simulink model "model_min_mine"  (R2018a)
settings: Solver=ode45  StartTime=0.0  StopTime=20  RelTol=1e-3
(part 2 of 10)

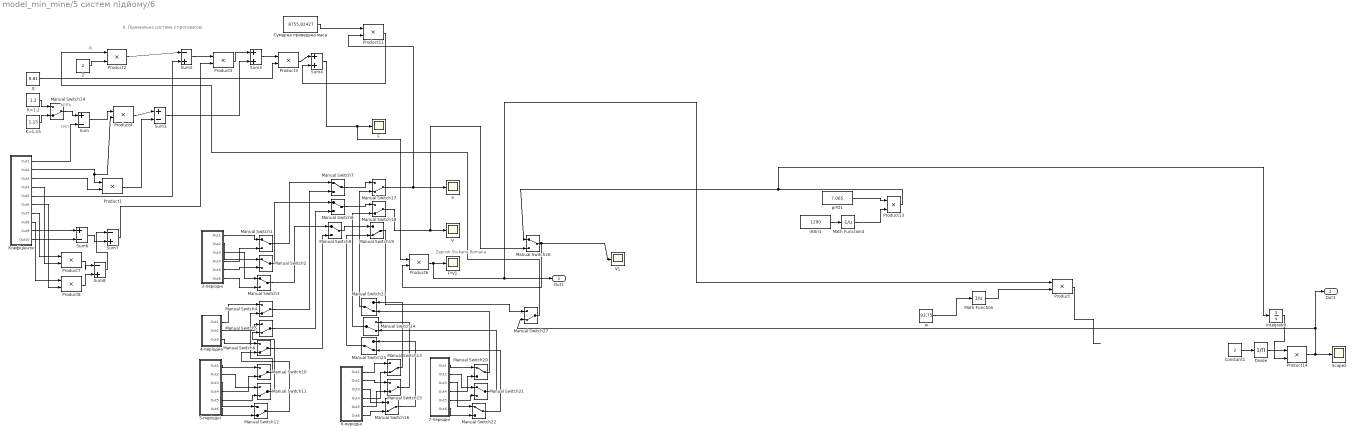
== system model_min_mine/5 систем підйому/6 ==
  note: кліть
  note: скіп
  note: Xi
  note: 6. Піднімальна система з противагою
  note: Zapusk Stukana Romana
  (60i)1 : Constant  Value=1200
  2 : Constant  Value=2
  3-періодні : Subsystem
  "4-періодна " : Subsystem
  5-періодні : Subsystem
  6-періодні : Subsystem
  7-періодні : Subsystem
  Constant1 : Constant  Value=2
  Divide : Product  Inputs=/
  F : Scope
  F*V1 : Scope
  Integrator : Integrator
  K=1.15 : Constant  Value=1.15
  K=1.2 : Constant  Value=1.2
  Manual Switch{1..3,7..9,20..22,26} (10 alike) : ManualSwitch
  Manual Switch{4..6,10..19,23..25,27} (17 alike) : ManualSwitch  CurrentSetting=0
  Math Function : Math  Operator=reciprocal  SaturateOnIntegerOverflow=on
  Math Function4 : Math  Operator=reciprocal  SaturateOnIntegerOverflow=on
  Product{,1..8,11,14} (11 alike) : Product  SaturateOnIntegerOverflow=on  OutDataTypeStr=Inherit: Same as first input
  Product13 : Product  Inputs=3  RndMeth=Zero
  Scope2 : Scope
  Sum : Sum  Inputs=|+-  SaturateOnIntegerOverflow=on
  Sum1 : Sum  Inputs=|+-  SaturateOnIntegerOverflow=on
  Sum2 : Sum  Inputs=|-+  SaturateOnIntegerOverflow=on
  Sum3 : Sum  Inputs=|++  SaturateOnIntegerOverflow=on
  Sum4 : Sum  Inputs=|++  SaturateOnIntegerOverflow=on
  Sum6 : Sum  Inputs=|+-  SaturateOnIntegerOverflow=on
  Sum7 : Sum  Inputs=|-+  SaturateOnIntegerOverflow=on
  Sum8 : Sum  Inputs=|-+  SaturateOnIntegerOverflow=on
  V : Scope
  V1 : Scope
  a : Scope
  g : Constant  Value=9.81
  pi*D1 : Constant  Value=7.065
  w : Constant  Value=93.75
  Коефіцієнти : Subsystem
  Сумарна приведена маса : Constant  Value=8755.82427
  Out1 : Outport
  Out3 : Outport  Port=2
  wires:
  K=1.2/1 -> Manual Switch14/1
  K=1.15/1 -> Manual Switch14/2
  Manual Switch14/1 -> Sum/1
  Коефіцієнти/1(Out1) -> Sum/2
  Sum/1 -> Product4/1
  Коефіцієнти/2(Out2) -> Product4/2, Product1/1
  Коефіцієнти/3(Out3) -> Product1/2
  Product4/1 -> Sum1/1
  Product1/1 -> Sum1/2
  Product2/1 -> Sum2/1
  Коефіцієнти/5(Out5) -> Sum2/2
  Sum1/1 -> Sum3/2
  Sum3/1 -> Product3/1
  g/1 -> Product3/2
  Коефіцієнти/4(Out4) -> Product7/2
  Sum2/1 -> Product5/1
  Product5/1 -> Sum3/1
  Product3/1 -> Sum4/1
  Sum4/1 -> F/1, Product6/1
  2/1 -> Product2/2
  Сумарна приведена маса/1 -> Product11/1
  Product11/1 -> Sum4/2
  Коефіцієнти/6(Out6) -> Product8/2
  Коефіцієнти/9(Out9) -> Sum6/1
  Коефіцієнти/10(Out10) -> Sum6/2
  Sum6/1 -> Sum7/2
  Коефіцієнти/7(Out7) -> Product7/1
  Коефіцієнти/8(Out8) -> Product8/1
  Product8/1 -> Sum8/2
  Product7/1 -> Sum8/1
  Sum8/1 -> Sum7/1
  Sum7/1 -> Product5/2
  Manual Switch25/1 -> Manual Switch19/2
  Manual Switch24/1 -> Manual Switch18/2
  Manual Switch23/1 -> Manual Switch17/2
  Manual Switch16/1 -> Manual Switch25/1
  Manual Switch15/1 -> Manual Switch24/1
  Manual Switch13/1 -> Manual Switch23/1
  Manual Switch22/1 -> Manual Switch25/2
  Manual Switch21/1 -> Manual Switch24/2
  Manual Switch20/1 -> Manual Switch23/2
  Manual Switch8/1 -> Manual Switch18/1
  Manual Switch17/1 -> a/1, Product11/2
  Manual Switch7/1 -> Manual Switch17/1
  Manual Switch12/1 -> Manual Switch6/2
  Manual Switch11/1 -> Manual Switch5/2
  Manual Switch10/1 -> Manual Switch4/2
  Manual Switch6/1 -> Manual Switch9/2
  Manual Switch5/1 -> Manual Switch8/2
  Manual Switch4/1 -> Manual Switch7/2
  Manual Switch9/1 -> Manual Switch19/1
  Manual Switch2/1 -> Manual Switch8/1
  Manual Switch1/1 -> Manual Switch7/1
  Manual Switch3/1 -> Manual Switch9/1
  Product6/1 -> F*V1/1, Out1/1, Product/1
  Manual Switch18/1 -> V/1, Manual Switch26/2
  3-періодні/1(Out1) -> Manual Switch1/1
  3-періодні/2(Out2) -> Manual Switch2/1
  3-періодні/3(Out3) -> Manual Switch3/1
  3-періодні/4(Out4) -> Manual Switch1/2
  3-періодні/5(Out5) -> Manual Switch2/2
  3-періодні/6(Out6) -> Manual Switch3/2
  "4-періодна "/1(Out1) -> Manual Switch4/1
  "4-періодна "/2(Out2) -> Manual Switch5/1
  "4-періодна "/3(Out3) -> Manual Switch6/1
  5-періодні/1(Out1) -> Manual Switch10/1
  5-періодні/2(Out2) -> Manual Switch11/1
  5-періодні/3(Out3) -> Manual Switch12/1
  5-періодні/4(Out4) -> Manual Switch10/2
  5-періодні/5(Out5) -> Manual Switch11/2
  5-періодні/6(Out6) -> Manual Switch12/2
  6-періодні/1(Out1) -> Manual Switch13/1
  6-періодні/2(Out2) -> Manual Switch15/1
  6-періодні/3(Out3) -> Manual Switch16/1
  6-періодні/4(Out4) -> Manual Switch13/2
  6-періодні/5(Out5) -> Manual Switch15/2
  6-періодні/6(Out6) -> Manual Switch16/2
  7-періодні/1(Out1) -> Manual Switch20/1
  7-періодні/2(Out2) -> Manual Switch21/1
  7-періодні/3(Out3) -> Manual Switch22/1
  7-періодні/4(Out4) -> Manual Switch20/2
  7-періодні/5(Out5) -> Manual Switch21/2
  7-періодні/6(Out6) -> Manual Switch22/2
  Product/1 -> ?
  Math Function/1 -> Product/2
  w/1 -> Math Function/1
  Integrator/1 -> Product14/2
  Product14/1 -> Scope2/1, Out3/1, Manual Switch27/2
  Divide/1 -> Product14/1
  Constant1/1 -> Divide/1
  pi*D1/1 -> Product13/1
  (60i)1/1 -> Math Function4/1
  Math Function4/1 -> Product13/3
  Product13/1 -> Manual Switch26/1, Integrator/1
  Manual Switch26/1 -> Product6/2, V1/1
  Manual Switch19/1 -> Manual Switch27/1
  Manual Switch27/1 -> Product2/1

== system model_min_mine/5 систем підйому/1/3-періодні ==
  note: 1. Криволінійна трьохперіодна
  note: a
  note: 2. Пр
  Криволінійна-3 : Subsystem
  Пр : Subsystem
  Out1 : Outport
  Out2 : Outport  Port=2
  Out3 : Outport  Port=3
  Out4 : Outport  Port=4
  Out5 : Outport  Port=5
  Out6 : Outport  Port=6
  wires:
  Криволінійна-3/1(Out1) -> Out1/1
  Криволінійна-3/2(Out2) -> Out2/1
  Криволінійна-3/3(Out3) -> Out3/1
  Пр/1(Out1) -> Out4/1
  Пр/2(Out2) -> Out5/1
  Пр/3(Out3) -> Out6/1

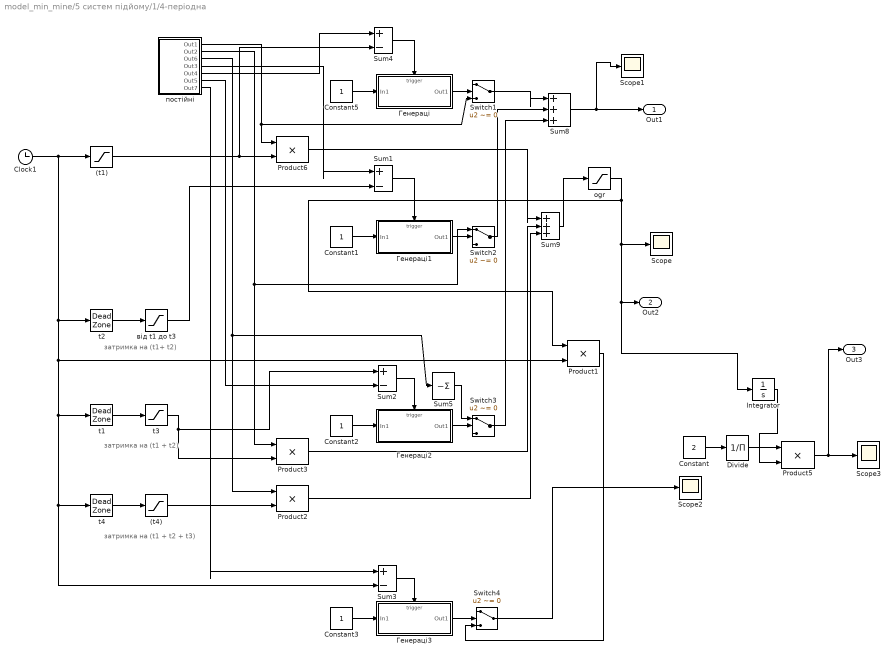
== system model_min_mine/5 систем підйому/1/4-періодна  ==
  note: затримка на
      | (t1 + t2 + t3)
  note: затримка на
      | (t1 + t2)
  note: затримка на
      |  (t1+ t2)
  (t1) : Saturate  UpperLimit=1.15  LowerLimit=0
  (t4) : Saturate  UpperLimit=1  LowerLimit=0
  Clock1 : Clock
  Constant : Constant  Value=2
  Constant{1..3,5} (4 alike) : Constant
  Divide : Product  Inputs=/
  Integrator : Integrator
  Product{1..3,5..6} (5 alike) : Product  SaturateOnIntegerOverflow=on  OutDataTypeStr=Inherit: Same as first input
  Scope{,1..3} (4 alike) : Scope
  Sum{1..4} (4 alike) : Sum  Inputs=|+-  SaturateOnIntegerOverflow=on
  Sum5 : Sum  Inputs=|-  SaturateOnIntegerOverflow=on
  Sum8 : Sum  Inputs=|+++  SaturateOnIntegerOverflow=on
  Sum9 : Sum  Inputs=|+++  SaturateOnIntegerOverflow=on
  Switch{1..4} (4 alike) : Switch  Criteria=u2 ~= 0  RndMeth=Zero  SaturateOnIntegerOverflow=on
  ogr : Saturate  UpperLimit=100  LowerLimit=0
  t1 : DeadZone  LowerValue=0  UpperValue=6.15  SaturateOnIntegerOverflow=on
  t2 : DeadZone  LowerValue=0  UpperValue=3.15  SaturateOnIntegerOverflow=on
  t3 : Saturate  UpperLimit=2  LowerLimit=0
  t4 : DeadZone  LowerValue=0  UpperValue=7.15  SaturateOnIntegerOverflow=on
  Генераці : Subsystem  TreatAsAtomicUnit=on
  Генераці1 : Subsystem  TreatAsAtomicUnit=on
  Генераці2 : Subsystem  TreatAsAtomicUnit=on
  Генераці3 : Subsystem  TreatAsAtomicUnit=on
  від t1 до t3 : Saturate  UpperLimit=3  LowerLimit=0
  постійні : Subsystem
  Out1 : Outport
  Out2 : Outport  Port=2
  Out3 : Outport  Port=3
  wires:
  (t4)/1 -> Product2/2
  t4/1 -> (t4)/1
  Product6/1 -> Sum9/1
  Product2/1 -> Sum9/3
  Product3/1 -> Sum9/2
  ogr/1 -> Product1/1, Scope/1, Out2/1, Integrator/1
  Sum5/1 -> Switch3/1
  від t1 до t3/1 -> Sum1/2
  Product1/1 -> Switch4/3
  Switch4/1 -> Scope2/1
  Генераці3/1(Out1) -> Switch4/2
  Sum3/1 -> Генераці3/Trigger
  Constant3/1 -> Генераці3/1(In1)
  постійні/7(Out7) -> Sum3/1
  t3/1 -> Product3/2, Sum2/1
  t1/1 -> t3/1
  постійні/6(Out5) -> Sum2/2
  Switch3/1 -> Sum8/3
  постійні/3(Out6) -> Sum5/1, Product2/1
  Constant2/1 -> Генераці2/1(In1)
  Sum2/1 -> Генераці2/Trigger
  Генераці2/1(Out1) -> Switch3/2
  постійні/1(Out1) -> Product6/1, Switch1/3
  t2/1 -> від t1 до t3/1
  Clock1/1 -> (t1)/1, t2/1, Product1/2, t1/1, Sum3/2, t4/1
  (t1)/1 -> Product6/2, Sum4/2
  постійні/2(Out2) -> Switch2/1, Product3/1
  Sum9/1 -> ogr/1
  Constant5/1 -> Генераці/1(In1)
  Sum4/1 -> Генераці/Trigger
  Генераці/1(Out1) -> Switch1/2
  Switch1/1 -> Sum8/1
  постійні/5(Out4) -> Sum4/1
  Constant1/1 -> Генераці1/1(In1)
  Sum1/1 -> Генераці1/Trigger
  Генераці1/1(Out1) -> Switch2/2
  постійні/4(Out3) -> Sum1/1
  Switch2/1 -> Sum8/2
  Sum8/1 -> Out1/1, Scope1/1
  Integrator/1 -> Product5/2
  Product5/1 -> Scope3/1, Out3/1
  Divide/1 -> Product5/1
  Constant/1 -> Divide/1

== system model_min_mine/5 систем підйому/1/5-періодні ==
  криво : Subsystem
  пр : Subsystem
  Out1 : Outport
  Out2 : Outport  Port=2
  Out3 : Outport  Port=3
  Out4 : Outport  Port=4
  Out5 : Outport  Port=5
  Out6 : Outport  Port=6
  wires:
  криво/1(Out1) -> Out1/1
  криво/2(Out2) -> Out2/1
  криво/3(Out3) -> Out3/1
  пр/1(Out1) -> Out4/1
  пр/2(Out2) -> Out5/1
  пр/3(Out3) -> Out6/1

== system model_min_mine/5 систем підйому/1/6-періодні ==
  6-ти періодна криволінійна : Subsystem
  6-ти періодна пр : Subsystem
  Out1 : Outport
  Out2 : Outport  Port=2
  Out3 : Outport  Port=3
  Out4 : Outport  Port=4
  Out5 : Outport  Port=5
  Out6 : Outport  Port=6
  wires:
  6-ти періодна криволінійна/1(Out1) -> Out1/1
  6-ти періодна криволінійна/2(Out2) -> Out2/1
  6-ти періодна криволінійна/3(Out3) -> Out3/1
  6-ти періодна пр/1(Out1) -> Out4/1
  6-ти періодна пр/2(Out2) -> Out5/1
  6-ти періодна пр/3(Out3) -> Out6/1

== system model_min_mine/5 систем підйому/1/7-періодні ==
  7-ми періодна криволінійна : Subsystem
  7-ми періодна пр : Subsystem
  Out1 : Outport
  Out2 : Outport  Port=2
  Out3 : Outport  Port=3
  Out4 : Outport  Port=4
  Out5 : Outport  Port=5
  Out6 : Outport  Port=6
  wires:
  7-ми періодна пр/1(Out1) -> Out1/1
  7-ми періодна пр/2(Out2) -> Out2/1
  7-ми періодна пр/3(Out3) -> Out3/1
  7-ми періодна криволінійна/1(Out1) -> Out4/1
  7-ми періодна криволінійна/2(Out2) -> Out5/1
  7-ми періодна криволінійна/3(Out3) -> Out6/1

== system model_min_mine/5 систем підйому/1/Коефіцієнти ==
  alfa : Constant  Value=1.15
  beta : Constant  Value=1.2
  m вантажу : Constant  Value=1000
  mк : Constant  Value=35
  "Висота стволу - Н, м" : Constant  Value=500
  Out1 : Outport
  Out2 : Outport  Port=2
  Out3 : Outport  Port=3
  Out4 : Outport  Port=4
  Out5 : Outport  Port=5
  wires:
  beta/1 -> Out1/1
  m вантажу/1 -> Out2/1
  alfa/1 -> Out3/1
  mк/1 -> Out4/1
  "Висота стволу - Н, м"/1 -> Out5/1

== system model_min_mine/5 систем підйому/2/3-періодні ==
  note: 1. Криволінійна трьохперіодна
  note: a
  note: 2. Пр
  Криволінійна-3 : Subsystem
  Пр : Subsystem
  Out1 : Outport
  Out2 : Outport  Port=2
  Out3 : Outport  Port=3
  Out4 : Outport  Port=4
  Out5 : Outport  Port=5
  Out6 : Outport  Port=6
  wires:
  Криволінійна-3/1(Out1) -> Out1/1
  Криволінійна-3/2(Out2) -> Out2/1
  Криволінійна-3/3(Out3) -> Out3/1
  Пр/1(Out1) -> Out4/1
  Пр/2(Out2) -> Out5/1
  Пр/3(Out3) -> Out6/1

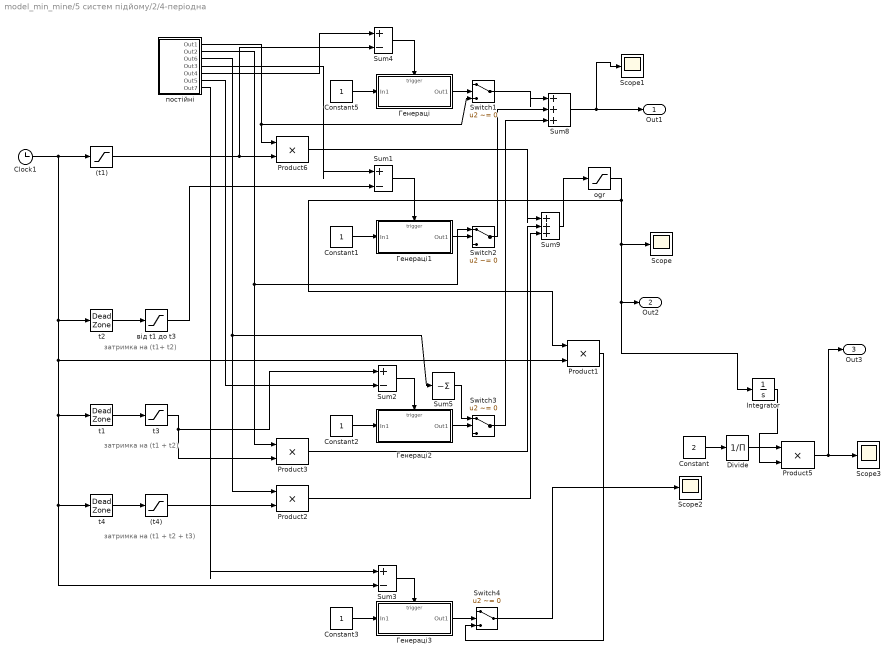
== system model_min_mine/5 систем підйому/2/4-періодна  ==
  note: затримка на
      | (t1 + t2 + t3)
  note: затримка на
      | (t1 + t2)
  note: затримка на
      |  (t1+ t2)
  (t1) : Saturate  UpperLimit=1.15  LowerLimit=0
  (t4) : Saturate  UpperLimit=1  LowerLimit=0
  Clock1 : Clock
  Constant : Constant  Value=2
  Constant{1..3,5} (4 alike) : Constant
  Divide : Product  Inputs=/
  Integrator : Integrator
  Product{1..3,5..6} (5 alike) : Product  SaturateOnIntegerOverflow=on  OutDataTypeStr=Inherit: Same as first input
  Scope{,1..3} (4 alike) : Scope
  Sum{1..4} (4 alike) : Sum  Inputs=|+-  SaturateOnIntegerOverflow=on
  Sum5 : Sum  Inputs=|-  SaturateOnIntegerOverflow=on
  Sum8 : Sum  Inputs=|+++  SaturateOnIntegerOverflow=on
  Sum9 : Sum  Inputs=|+++  SaturateOnIntegerOverflow=on
  Switch{1..4} (4 alike) : Switch  Criteria=u2 ~= 0  RndMeth=Zero  SaturateOnIntegerOverflow=on
  ogr : Saturate  UpperLimit=100  LowerLimit=0
  t1 : DeadZone  LowerValue=0  UpperValue=6.15  SaturateOnIntegerOverflow=on
  t2 : DeadZone  LowerValue=0  UpperValue=3.15  SaturateOnIntegerOverflow=on
  t3 : Saturate  UpperLimit=2  LowerLimit=0
  t4 : DeadZone  LowerValue=0  UpperValue=7.15  SaturateOnIntegerOverflow=on
  Генераці : Subsystem  TreatAsAtomicUnit=on
  Генераці1 : Subsystem  TreatAsAtomicUnit=on
  Генераці2 : Subsystem  TreatAsAtomicUnit=on
  Генераці3 : Subsystem  TreatAsAtomicUnit=on
  від t1 до t3 : Saturate  UpperLimit=3  LowerLimit=0
  постійні : Subsystem
  Out1 : Outport
  Out2 : Outport  Port=2
  Out3 : Outport  Port=3
  wires:
  (t4)/1 -> Product2/2
  t4/1 -> (t4)/1
  Product6/1 -> Sum9/1
  Product2/1 -> Sum9/3
  Product3/1 -> Sum9/2
  ogr/1 -> Product1/1, Scope/1, Out2/1, Integrator/1
  Sum5/1 -> Switch3/1
  від t1 до t3/1 -> Sum1/2
  Product1/1 -> Switch4/3
  Switch4/1 -> Scope2/1
  Генераці3/1(Out1) -> Switch4/2
  Sum3/1 -> Генераці3/Trigger
  Constant3/1 -> Генераці3/1(In1)
  постійні/7(Out7) -> Sum3/1
  t3/1 -> Product3/2, Sum2/1
  t1/1 -> t3/1
  постійні/6(Out5) -> Sum2/2
  Switch3/1 -> Sum8/3
  постійні/3(Out6) -> Sum5/1, Product2/1
  Constant2/1 -> Генераці2/1(In1)
  Sum2/1 -> Генераці2/Trigger
  Генераці2/1(Out1) -> Switch3/2
  постійні/1(Out1) -> Product6/1, Switch1/3
  t2/1 -> від t1 до t3/1
  Clock1/1 -> (t1)/1, t2/1, Product1/2, t1/1, Sum3/2, t4/1
  (t1)/1 -> Product6/2, Sum4/2
  постійні/2(Out2) -> Switch2/1, Product3/1
  Sum9/1 -> ogr/1
  Constant5/1 -> Генераці/1(In1)
  Sum4/1 -> Генераці/Trigger
  Генераці/1(Out1) -> Switch1/2
  Switch1/1 -> Sum8/1
  постійні/5(Out4) -> Sum4/1
  Constant1/1 -> Генераці1/1(In1)
  Sum1/1 -> Генераці1/Trigger
  Генераці1/1(Out1) -> Switch2/2
  постійні/4(Out3) -> Sum1/1
  Switch2/1 -> Sum8/2
  Sum8/1 -> Out1/1, Scope1/1
  Integrator/1 -> Product5/2
  Product5/1 -> Scope3/1, Out3/1
  Divide/1 -> Product5/1
  Constant/1 -> Divide/1

== system model_min_mine/5 систем підйому/2/5-періодні ==
  криво : Subsystem
  пр : Subsystem
  Out1 : Outport
  Out2 : Outport  Port=2
  Out3 : Outport  Port=3
  Out4 : Outport  Port=4
  Out5 : Outport  Port=5
  Out6 : Outport  Port=6
  wires:
  криво/1(Out1) -> Out1/1
  криво/2(Out2) -> Out2/1
  криво/3(Out3) -> Out3/1
  пр/1(Out1) -> Out4/1
  пр/2(Out2) -> Out5/1
  пр/3(Out3) -> Out6/1

== system model_min_mine/5 систем підйому/2/6-періодні ==
  6-ти періодна криволінійна : Subsystem
  6-ти періодна пр : Subsystem
  Out1 : Outport
  Out2 : Outport  Port=2
  Out3 : Outport  Port=3
  Out4 : Outport  Port=4
  Out5 : Outport  Port=5
  Out6 : Outport  Port=6
  wires:
  6-ти періодна криволінійна/1(Out1) -> Out1/1
  6-ти періодна криволінійна/2(Out2) -> Out2/1
  6-ти періодна криволінійна/3(Out3) -> Out3/1
  6-ти періодна пр/1(Out1) -> Out4/1
  6-ти періодна пр/2(Out2) -> Out5/1
  6-ти періодна пр/3(Out3) -> Out6/1

== system model_min_mine/5 систем підйому/2/7-періодні ==
  7-ми періодна криволінійна : Subsystem
  7-ми періодна пр : Subsystem
  Out1 : Outport
  Out2 : Outport  Port=2
  Out3 : Outport  Port=3
  Out4 : Outport  Port=4
  Out5 : Outport  Port=5
  Out6 : Outport  Port=6
  wires:
  7-ми періодна пр/1(Out1) -> Out1/1
  7-ми періодна пр/2(Out2) -> Out2/1
  7-ми періодна пр/3(Out3) -> Out3/1
  7-ми періодна криволінійна/1(Out1) -> Out4/1
  7-ми періодна криволінійна/2(Out2) -> Out5/1
  7-ми періодна криволінійна/3(Out3) -> Out6/1

== system model_min_mine/5 систем підйому/2/Коефіцієнти ==
  alfa : Constant  Value=1.15
  beta : Constant  Value=1.2
  m вантажу : Constant  Value=1000
  Out1 : Outport
  Out2 : Outport  Port=2
  Out3 : Outport  Port=3
  wires:
  beta/1 -> Out1/1
  m вантажу/1 -> Out2/1
  alfa/1 -> Out3/1

== system model_min_mine/5 систем підйому/3/3-періодні ==
  note: 1. Криволінійна трьохперіодна
  note: a
  note: 2. Пр
  Криволінійна-3 : Subsystem
  Пр : Subsystem
  Out1 : Outport
  Out2 : Outport  Port=2
  Out3 : Outport  Port=3
  Out4 : Outport  Port=4
  Out5 : Outport  Port=5
  Out6 : Outport  Port=6
  wires:
  Криволінійна-3/1(Out1) -> Out1/1
  Криволінійна-3/2(Out2) -> Out2/1
  Криволінійна-3/3(Out3) -> Out3/1
  Пр/1(Out1) -> Out4/1
  Пр/2(Out2) -> Out5/1
  Пр/3(Out3) -> Out6/1

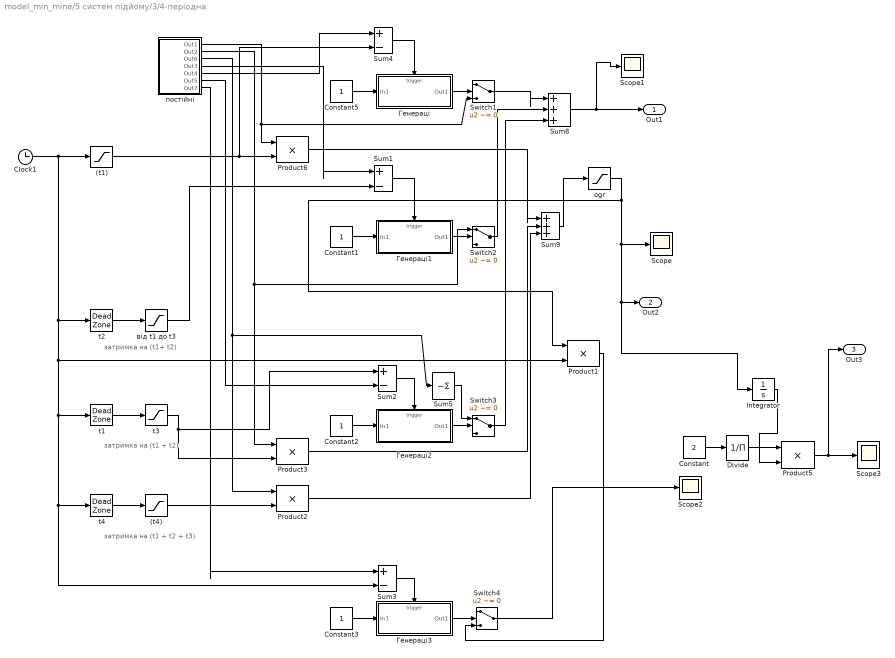
== system model_min_mine/5 систем підйому/3/4-періодна  ==
  note: затримка на
      | (t1 + t2 + t3)
  note: затримка на
      | (t1 + t2)
  note: затримка на
      |  (t1+ t2)
  (t1) : Saturate  UpperLimit=1.15  LowerLimit=0
  (t4) : Saturate  UpperLimit=1  LowerLimit=0
  Clock1 : Clock
  Constant : Constant  Value=2
  Constant{1..3,5} (4 alike) : Constant
  Divide : Product  Inputs=/
  Integrator : Integrator
  Product{1..3,5..6} (5 alike) : Product  SaturateOnIntegerOverflow=on  OutDataTypeStr=Inherit: Same as first input
  Scope{,1..3} (4 alike) : Scope
  Sum{1..4} (4 alike) : Sum  Inputs=|+-  SaturateOnIntegerOverflow=on
  Sum5 : Sum  Inputs=|-  SaturateOnIntegerOverflow=on
  Sum8 : Sum  Inputs=|+++  SaturateOnIntegerOverflow=on
  Sum9 : Sum  Inputs=|+++  SaturateOnIntegerOverflow=on
  Switch{1..4} (4 alike) : Switch  Criteria=u2 ~= 0  RndMeth=Zero  SaturateOnIntegerOverflow=on
  ogr : Saturate  UpperLimit=100  LowerLimit=0
  t1 : DeadZone  LowerValue=0  UpperValue=6.15  SaturateOnIntegerOverflow=on
  t2 : DeadZone  LowerValue=0  UpperValue=3.15  SaturateOnIntegerOverflow=on
  t3 : Saturate  UpperLimit=2  LowerLimit=0
  t4 : DeadZone  LowerValue=0  UpperValue=7.15  SaturateOnIntegerOverflow=on
  Генераці : Subsystem  TreatAsAtomicUnit=on
  Генераці1 : Subsystem  TreatAsAtomicUnit=on
  Генераці2 : Subsystem  TreatAsAtomicUnit=on
  Генераці3 : Subsystem  TreatAsAtomicUnit=on
  від t1 до t3 : Saturate  UpperLimit=3  LowerLimit=0
  постійні : Subsystem
  Out1 : Outport
  Out2 : Outport  Port=2
  Out3 : Outport  Port=3
  wires:
  (t4)/1 -> Product2/2
  t4/1 -> (t4)/1
  Product6/1 -> Sum9/1
  Product2/1 -> Sum9/3
  Product3/1 -> Sum9/2
  ogr/1 -> Product1/1, Scope/1, Out2/1, Integrator/1
  Sum5/1 -> Switch3/1
  від t1 до t3/1 -> Sum1/2
  Product1/1 -> Switch4/3
  Switch4/1 -> Scope2/1
  Генераці3/1(Out1) -> Switch4/2
  Sum3/1 -> Генераці3/Trigger
  Constant3/1 -> Генераці3/1(In1)
  постійні/7(Out7) -> Sum3/1
  t3/1 -> Product3/2, Sum2/1
  t1/1 -> t3/1
  постійні/6(Out5) -> Sum2/2
  Switch3/1 -> Sum8/3
  постійні/3(Out6) -> Sum5/1, Product2/1
  Constant2/1 -> Генераці2/1(In1)
  Sum2/1 -> Генераці2/Trigger
  Генераці2/1(Out1) -> Switch3/2
  постійні/1(Out1) -> Product6/1, Switch1/3
  t2/1 -> від t1 до t3/1
  Clock1/1 -> (t1)/1, t2/1, Product1/2, t1/1, Sum3/2, t4/1
  (t1)/1 -> Product6/2, Sum4/2
  постійні/2(Out2) -> Switch2/1, Product3/1
  Sum9/1 -> ogr/1
  Constant5/1 -> Генераці/1(In1)
  Sum4/1 -> Генераці/Trigger
  Генераці/1(Out1) -> Switch1/2
  Switch1/1 -> Sum8/1
  постійні/5(Out4) -> Sum4/1
  Constant1/1 -> Генераці1/1(In1)
  Sum1/1 -> Генераці1/Trigger
  Генераці1/1(Out1) -> Switch2/2
  постійні/4(Out3) -> Sum1/1
  Switch2/1 -> Sum8/2
  Sum8/1 -> Out1/1, Scope1/1
  Integrator/1 -> Product5/2
  Product5/1 -> Scope3/1, Out3/1
  Divide/1 -> Product5/1
  Constant/1 -> Divide/1

== system model_min_mine/5 систем підйому/3/5-періодні ==
  криво : Subsystem
  пр : Subsystem
  Out1 : Outport
  Out2 : Outport  Port=2
  Out3 : Outport  Port=3
  Out4 : Outport  Port=4
  Out5 : Outport  Port=5
  Out6 : Outport  Port=6
  wires:
  криво/1(Out1) -> Out1/1
  криво/2(Out2) -> Out2/1
  криво/3(Out3) -> Out3/1
  пр/1(Out1) -> Out4/1
  пр/2(Out2) -> Out5/1
  пр/3(Out3) -> Out6/1

== system model_min_mine/5 систем підйому/3/6-періодні ==
  6-ти періодна криволінійна : Subsystem
  6-ти періодна пр : Subsystem
  Out1 : Outport
  Out2 : Outport  Port=2
  Out3 : Outport  Port=3
  Out4 : Outport  Port=4
  Out5 : Outport  Port=5
  Out6 : Outport  Port=6
  wires:
  6-ти періодна криволінійна/1(Out1) -> Out1/1
  6-ти періодна криволінійна/2(Out2) -> Out2/1
  6-ти періодна криволінійна/3(Out3) -> Out3/1
  6-ти періодна пр/1(Out1) -> Out4/1
  6-ти періодна пр/2(Out2) -> Out5/1
  6-ти періодна пр/3(Out3) -> Out6/1

== system model_min_mine/5 систем підйому/3/7-періодні ==
  7-ми періодна криволінійна : Subsystem
  7-ми періодна пр : Subsystem
  Out1 : Outport
  Out2 : Outport  Port=2
  Out3 : Outport  Port=3
  Out4 : Outport  Port=4
  Out5 : Outport  Port=5
  Out6 : Outport  Port=6
  wires:
  7-ми періодна пр/1(Out1) -> Out1/1
  7-ми періодна пр/2(Out2) -> Out2/1
  7-ми періодна пр/3(Out3) -> Out3/1
  7-ми періодна криволінійна/1(Out1) -> Out4/1
  7-ми періодна криволінійна/2(Out2) -> Out5/1
  7-ми періодна криволінійна/3(Out3) -> Out6/1

== system model_min_mine/5 систем підйому/3/Коефіцієнти ==
  alfa : Constant  Value=1.15
  beta : Constant  Value=1.2
  m вантажу : Constant  Value=1000
  mк : Constant  Value=35
  "mк/ " : Constant  Value=45
  "Висота стволу - Н, м" : Constant  Value=500
  Out1 : Outport
  Out2 : Outport  Port=2
  Out3 : Outport  Port=3
  Out4 : Outport  Port=4
  Out5 : Outport  Port=5
  Out6 : Outport  Port=6
  wires:
  beta/1 -> Out1/1
  m вантажу/1 -> Out2/1
  alfa/1 -> Out3/1
  mк/1 -> Out4/1
  "Висота стволу - Н, м"/1 -> Out5/1
  "mк/ "/1 -> Out6/1

== system model_min_mine/5 систем підйому/4/3-періодні ==
  note: 1. Криволінійна трьохперіодна
  note: a
  note: 2. Пр
  Криволінійна-3 : Subsystem
  Пр : Subsystem
  Out1 : Outport
  Out2 : Outport  Port=2
  Out3 : Outport  Port=3
  Out4 : Outport  Port=4
  Out5 : Outport  Port=5
  Out6 : Outport  Port=6
  wires:
  Криволінійна-3/1(Out1) -> Out1/1
  Криволінійна-3/2(Out2) -> Out2/1
  Криволінійна-3/3(Out3) -> Out3/1
  Пр/1(Out1) -> Out4/1
  Пр/2(Out2) -> Out5/1
  Пр/3(Out3) -> Out6/1

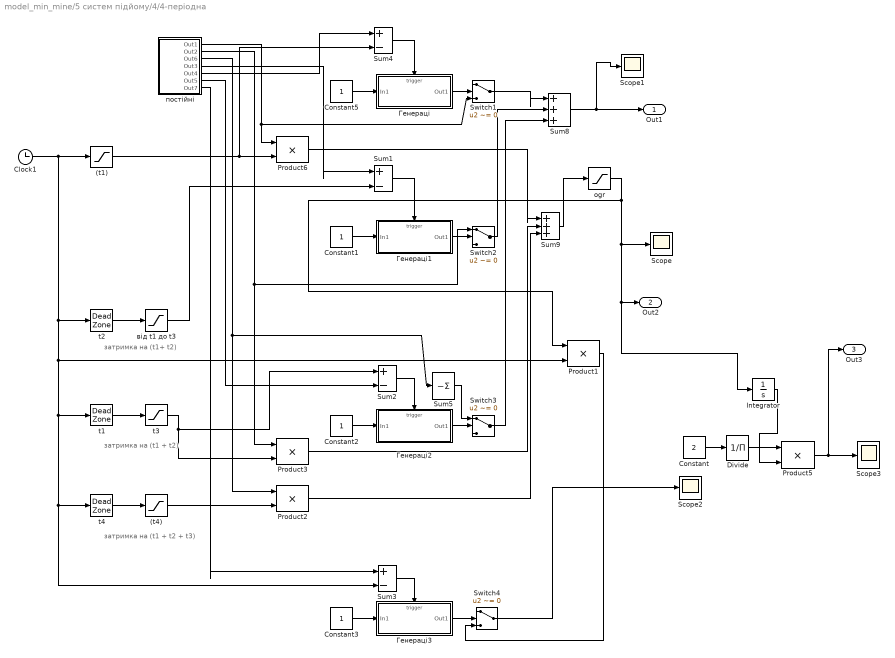
== system model_min_mine/5 систем підйому/4/4-періодна  ==
  note: затримка на
      | (t1 + t2 + t3)
  note: затримка на
      | (t1 + t2)
  note: затримка на
      |  (t1+ t2)
  (t1) : Saturate  UpperLimit=1.15  LowerLimit=0
  (t4) : Saturate  UpperLimit=1  LowerLimit=0
  Clock1 : Clock
  Constant : Constant  Value=2
  Constant{1..3,5} (4 alike) : Constant
  Divide : Product  Inputs=/
  Integrator : Integrator
  Product{1..3,5..6} (5 alike) : Product  SaturateOnIntegerOverflow=on  OutDataTypeStr=Inherit: Same as first input
  Scope{,1..3} (4 alike) : Scope
  Sum{1..4} (4 alike) : Sum  Inputs=|+-  SaturateOnIntegerOverflow=on
  Sum5 : Sum  Inputs=|-  SaturateOnIntegerOverflow=on
  Sum8 : Sum  Inputs=|+++  SaturateOnIntegerOverflow=on
  Sum9 : Sum  Inputs=|+++  SaturateOnIntegerOverflow=on
  Switch{1..4} (4 alike) : Switch  Criteria=u2 ~= 0  RndMeth=Zero  SaturateOnIntegerOverflow=on
  ogr : Saturate  UpperLimit=100  LowerLimit=0
  t1 : DeadZone  LowerValue=0  UpperValue=6.15  SaturateOnIntegerOverflow=on
  t2 : DeadZone  LowerValue=0  UpperValue=3.15  SaturateOnIntegerOverflow=on
  t3 : Saturate  UpperLimit=2  LowerLimit=0
  t4 : DeadZone  LowerValue=0  UpperValue=7.15  SaturateOnIntegerOverflow=on
  Генераці : Subsystem  TreatAsAtomicUnit=on
  Генераці1 : Subsystem  TreatAsAtomicUnit=on
  Генераці2 : Subsystem  TreatAsAtomicUnit=on
  Генераці3 : Subsystem  TreatAsAtomicUnit=on
  від t1 до t3 : Saturate  UpperLimit=3  LowerLimit=0
  постійні : Subsystem
  Out1 : Outport
  Out2 : Outport  Port=2
  Out3 : Outport  Port=3
  wires:
  (t4)/1 -> Product2/2
  t4/1 -> (t4)/1
  Product6/1 -> Sum9/1
  Product2/1 -> Sum9/3
  Product3/1 -> Sum9/2
  ogr/1 -> Product1/1, Scope/1, Out2/1, Integrator/1
  Sum5/1 -> Switch3/1
  від t1 до t3/1 -> Sum1/2
  Product1/1 -> Switch4/3
  Switch4/1 -> Scope2/1
  Генераці3/1(Out1) -> Switch4/2
  Sum3/1 -> Генераці3/Trigger
  Constant3/1 -> Генераці3/1(In1)
  постійні/7(Out7) -> Sum3/1
  t3/1 -> Product3/2, Sum2/1
  t1/1 -> t3/1
  постійні/6(Out5) -> Sum2/2
  Switch3/1 -> Sum8/3
  постійні/3(Out6) -> Sum5/1, Product2/1
  Constant2/1 -> Генераці2/1(In1)
  Sum2/1 -> Генераці2/Trigger
  Генераці2/1(Out1) -> Switch3/2
  постійні/1(Out1) -> Product6/1, Switch1/3
  t2/1 -> від t1 до t3/1
  Clock1/1 -> (t1)/1, t2/1, Product1/2, t1/1, Sum3/2, t4/1
  (t1)/1 -> Product6/2, Sum4/2
  постійні/2(Out2) -> Switch2/1, Product3/1
  Sum9/1 -> ogr/1
  Constant5/1 -> Генераці/1(In1)
  Sum4/1 -> Генераці/Trigger
  Генераці/1(Out1) -> Switch1/2
  Switch1/1 -> Sum8/1
  постійні/5(Out4) -> Sum4/1
  Constant1/1 -> Генераці1/1(In1)
  Sum1/1 -> Генераці1/Trigger
  Генераці1/1(Out1) -> Switch2/2
  постійні/4(Out3) -> Sum1/1
  Switch2/1 -> Sum8/2
  Sum8/1 -> Out1/1, Scope1/1
  Integrator/1 -> Product5/2
  Product5/1 -> Scope3/1, Out3/1
  Divide/1 -> Product5/1
  Constant/1 -> Divide/1

== system model_min_mine/5 систем підйому/4/5-періодні ==
  криво : Subsystem
  пр : Subsystem
  Out1 : Outport
  Out2 : Outport  Port=2
  Out3 : Outport  Port=3
  Out4 : Outport  Port=4
  Out5 : Outport  Port=5
  Out6 : Outport  Port=6
  wires:
  криво/1(Out1) -> Out1/1
  криво/2(Out2) -> Out2/1
  криво/3(Out3) -> Out3/1
  пр/1(Out1) -> Out4/1
  пр/2(Out2) -> Out5/1
  пр/3(Out3) -> Out6/1

== system model_min_mine/5 систем підйому/4/6-періодні ==
  6-ти періодна криволінійна : Subsystem
  6-ти періодна пр : Subsystem
  Out1 : Outport
  Out2 : Outport  Port=2
  Out3 : Outport  Port=3
  Out4 : Outport  Port=4
  Out5 : Outport  Port=5
  Out6 : Outport  Port=6
  wires:
  6-ти періодна криволінійна/1(Out1) -> Out1/1
  6-ти періодна криволінійна/2(Out2) -> Out2/1
  6-ти періодна криволінійна/3(Out3) -> Out3/1
  6-ти періодна пр/1(Out1) -> Out4/1
  6-ти періодна пр/2(Out2) -> Out5/1
  6-ти періодна пр/3(Out3) -> Out6/1

== system model_min_mine/5 систем підйому/4/7-періодні ==
  7-ми періодна криволінійна : Subsystem
  7-ми періодна пр : Subsystem
  Out1 : Outport
  Out2 : Outport  Port=2
  Out3 : Outport  Port=3
  Out4 : Outport  Port=4
  Out5 : Outport  Port=5
  Out6 : Outport  Port=6
  wires:
  7-ми періодна пр/1(Out1) -> Out1/1
  7-ми періодна пр/2(Out2) -> Out2/1
  7-ми періодна пр/3(Out3) -> Out3/1
  7-ми періодна криволінійна/1(Out1) -> Out4/1
  7-ми періодна криволінійна/2(Out2) -> Out5/1
  7-ми періодна криволінійна/3(Out3) -> Out6/1

== system model_min_mine/5 систем підйому/4/Коефіцієнти ==
  Z1 : Constant  Value=2
  Z2 : Constant  Value=3
  alfa : Constant  Value=1.15
  beta : Constant  Value=1.2
  m вантажу : Constant  Value=1000
  m противаги : Constant  Value=10000
  m скіпа : Constant  Value=15000
  mк : Constant  Value=35
  "mк/ " : Constant  Value=45
  "Висота стволу - Н, м" : Constant  Value=500
  Out1 : Outport
  Out2 : Outport  Port=2
  Out3 : Outport  Port=3
  Out4 : Outport  Port=4
  Out5 : Outport  Port=5
  Out6 : Outport  Port=6
  Out7 : Outport  Port=7
  Out8 : Outport  Port=8
  Out9 : Outport  Port=9
  Out10 : Outport  Port=10
  wires:
  beta/1 -> Out1/1
  m вантажу/1 -> Out2/1
  alfa/1 -> Out3/1
  mк/1 -> Out4/1
  "Висота стволу - Н, м"/1 -> Out5/1
  "mк/ "/1 -> Out6/1
  Z1/1 -> Out7/1
  Z2/1 -> Out8/1
  m скіпа/1 -> Out9/1
  m противаги/1 -> Out10/1

== system model_min_mine/5 систем підйому/6/3-періодні ==
  note: 1. Криволінійна трьохперіодна
  note: a
  note: 2. Пр
  Криволінійна-3 : Subsystem
  Пр : Subsystem
  Out1 : Outport
  Out2 : Outport  Port=2
  Out3 : Outport  Port=3
  Out4 : Outport  Port=4
  Out5 : Outport  Port=5
  Out6 : Outport  Port=6
  wires:
  Криволінійна-3/1(Out1) -> Out1/1
  Криволінійна-3/2(Out2) -> Out2/1
  Криволінійна-3/3(Out3) -> Out3/1
  Пр/1(Out1) -> Out4/1
  Пр/2(Out2) -> Out5/1
  Пр/3(Out3) -> Out6/1

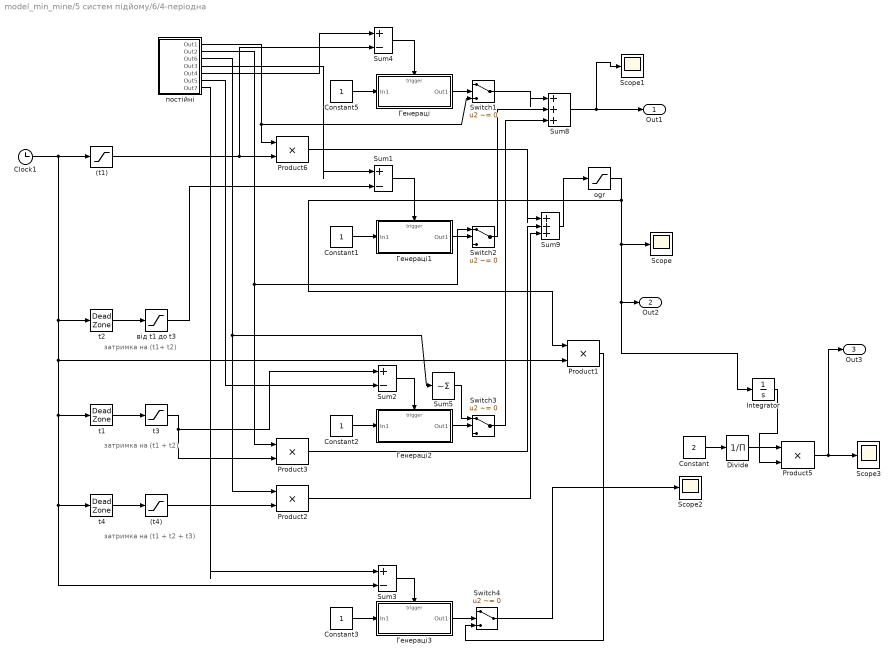
== system model_min_mine/5 систем підйому/6/4-періодна  ==
  note: затримка на
      | (t1 + t2 + t3)
  note: затримка на
      | (t1 + t2)
  note: затримка на
      |  (t1+ t2)
  (t1) : Saturate  UpperLimit=1.15  LowerLimit=0
  (t4) : Saturate  UpperLimit=1  LowerLimit=0
  Clock1 : Clock
  Constant : Constant  Value=2
  Constant{1..3,5} (4 alike) : Constant
  Divide : Product  Inputs=/
  Integrator : Integrator
  Product{1..3,5..6} (5 alike) : Product  SaturateOnIntegerOverflow=on  OutDataTypeStr=Inherit: Same as first input
  Scope{,1..3} (4 alike) : Scope
  Sum{1..4} (4 alike) : Sum  Inputs=|+-  SaturateOnIntegerOverflow=on
  Sum5 : Sum  Inputs=|-  SaturateOnIntegerOverflow=on
  Sum8 : Sum  Inputs=|+++  SaturateOnIntegerOverflow=on
  Sum9 : Sum  Inputs=|+++  SaturateOnIntegerOverflow=on
  Switch{1..4} (4 alike) : Switch  Criteria=u2 ~= 0  RndMeth=Zero  SaturateOnIntegerOverflow=on
  ogr : Saturate  UpperLimit=100  LowerLimit=0
  t1 : DeadZone  LowerValue=0  UpperValue=6.15  SaturateOnIntegerOverflow=on
  t2 : DeadZone  LowerValue=0  UpperValue=3.15  SaturateOnIntegerOverflow=on
  t3 : Saturate  UpperLimit=2  LowerLimit=0
  t4 : DeadZone  LowerValue=0  UpperValue=7.15  SaturateOnIntegerOverflow=on
  Генераці : Subsystem  TreatAsAtomicUnit=on
  Генераці1 : Subsystem  TreatAsAtomicUnit=on
  Генераці2 : Subsystem  TreatAsAtomicUnit=on
  Генераці3 : Subsystem  TreatAsAtomicUnit=on
  від t1 до t3 : Saturate  UpperLimit=3  LowerLimit=0
  постійні : Subsystem
  Out1 : Outport
  Out2 : Outport  Port=2
  Out3 : Outport  Port=3
  wires:
  (t4)/1 -> Product2/2
  t4/1 -> (t4)/1
  Product6/1 -> Sum9/1
  Product2/1 -> Sum9/3
  Product3/1 -> Sum9/2
  ogr/1 -> Product1/1, Scope/1, Out2/1, Integrator/1
  Sum5/1 -> Switch3/1
  від t1 до t3/1 -> Sum1/2
  Product1/1 -> Switch4/3
  Switch4/1 -> Scope2/1
  Генераці3/1(Out1) -> Switch4/2
  Sum3/1 -> Генераці3/Trigger
  Constant3/1 -> Генераці3/1(In1)
  постійні/7(Out7) -> Sum3/1
  t3/1 -> Product3/2, Sum2/1
  t1/1 -> t3/1
  постійні/6(Out5) -> Sum2/2
  Switch3/1 -> Sum8/3
  постійні/3(Out6) -> Sum5/1, Product2/1
  Constant2/1 -> Генераці2/1(In1)
  Sum2/1 -> Генераці2/Trigger
  Генераці2/1(Out1) -> Switch3/2
  постійні/1(Out1) -> Product6/1, Switch1/3
  t2/1 -> від t1 до t3/1
  Clock1/1 -> (t1)/1, t2/1, Product1/2, t1/1, Sum3/2, t4/1
  (t1)/1 -> Product6/2, Sum4/2
  постійні/2(Out2) -> Switch2/1, Product3/1
  Sum9/1 -> ogr/1
  Constant5/1 -> Генераці/1(In1)
  Sum4/1 -> Генераці/Trigger
  Генераці/1(Out1) -> Switch1/2
  Switch1/1 -> Sum8/1
  постійні/5(Out4) -> Sum4/1
  Constant1/1 -> Генераці1/1(In1)
  Sum1/1 -> Генераці1/Trigger
  Генераці1/1(Out1) -> Switch2/2
  постійні/4(Out3) -> Sum1/1
  Switch2/1 -> Sum8/2
  Sum8/1 -> Out1/1, Scope1/1
  Integrator/1 -> Product5/2
  Product5/1 -> Scope3/1, Out3/1
  Divide/1 -> Product5/1
  Constant/1 -> Divide/1

== system model_min_mine/5 систем підйому/6/5-періодні ==
  криво : Subsystem
  пр : Subsystem
  Out1 : Outport
  Out2 : Outport  Port=2
  Out3 : Outport  Port=3
  Out4 : Outport  Port=4
  Out5 : Outport  Port=5
  Out6 : Outport  Port=6
  wires:
  криво/1(Out1) -> Out1/1
  криво/2(Out2) -> Out2/1
  криво/3(Out3) -> Out3/1
  пр/1(Out1) -> Out4/1
  пр/2(Out2) -> Out5/1
  пр/3(Out3) -> Out6/1

== system model_min_mine/5 систем підйому/6/6-періодні ==
  6-ти періодна криволінійна : Subsystem
  6-ти періодна пр : Subsystem
  Out1 : Outport
  Out2 : Outport  Port=2
  Out3 : Outport  Port=3
  Out4 : Outport  Port=4
  Out5 : Outport  Port=5
  Out6 : Outport  Port=6
  wires:
  6-ти періодна криволінійна/1(Out1) -> Out1/1
  6-ти періодна криволінійна/2(Out2) -> Out2/1
  6-ти періодна криволінійна/3(Out3) -> Out3/1
  6-ти періодна пр/1(Out1) -> Out4/1
  6-ти періодна пр/2(Out2) -> Out5/1
  6-ти періодна пр/3(Out3) -> Out6/1

== system model_min_mine/5 систем підйому/6/7-періодні ==
  7-ми періодна криволінійна : Subsystem
  7-ми періодна пр : Subsystem
  Out1 : Outport
  Out2 : Outport  Port=2
  Out3 : Outport  Port=3
  Out4 : Outport  Port=4
  Out5 : Outport  Port=5
  Out6 : Outport  Port=6
  wires:
  7-ми періодна пр/1(Out1) -> Out1/1
  7-ми періодна пр/2(Out2) -> Out2/1
  7-ми періодна пр/3(Out3) -> Out3/1
  7-ми періодна криволінійна/1(Out1) -> Out4/1
  7-ми періодна криволінійна/2(Out2) -> Out5/1
  7-ми періодна криволінійна/3(Out3) -> Out6/1

== system model_min_mine/5 систем підйому/6/Коефіцієнти ==
  Z1 : Constant  Value=2
  Z2 : Constant  Value=3
  alfa : Constant  Value=1.15
  beta : Constant  Value=1.2
  m вантажу : Constant  Value=12000
  m противаги : Constant  Value=12670
  m скіпа : Constant  Value=12670
  mк : Constant  Value=3.5
  "mк/ " : Constant  Value=4.5
  "Висота стволу - Н, м" : Constant  Value=880
  Out1 : Outport
  Out2 : Outport  Port=2
  Out3 : Outport  Port=3
  Out4 : Outport  Port=4
  Out5 : Outport  Port=5
  Out6 : Outport  Port=6
  Out7 : Outport  Port=7
  Out8 : Outport  Port=8
  Out9 : Outport  Port=9
  Out10 : Outport  Port=10
  wires:
  beta/1 -> Out1/1
  m вантажу/1 -> Out2/1
  alfa/1 -> Out3/1
  mк/1 -> Out4/1
  "Висота стволу - Н, м"/1 -> Out5/1
  "mк/ "/1 -> Out6/1
  Z1/1 -> Out7/1
  Z2/1 -> Out8/1
  m скіпа/1 -> Out9/1
  m противаги/1 -> Out10/1

== system model_min_mine/5 систем підйому/1/3-періодні/Криволінійна-3 ==
  (t1) : Saturate  UpperLimit=1.15  LowerLimit=0
  (t1+ t2) : DeadZone  LowerValue=0  UpperValue=3.15  SaturateOnIntegerOverflow=on
  Clock1 : Clock
  Constant : Constant  Value=2
  Constant1 : Constant
  Divide : Product  Inputs=/
  Integrator : Integrator
  Product5 : Product  SaturateOnIntegerOverflow=on  OutDataTypeStr=Inherit: Same as first input
  Scope2 : Scope
  Sum1 : Sum  Inputs=|+-  SaturateOnIntegerOverflow=on
  Sum8 : Sum  Inputs=|++  SaturateOnIntegerOverflow=on
  Sum9 : Sum  Inputs=|++  SaturateOnIntegerOverflow=on
  Switch2 : Switch  Criteria=u2 ~= 0  RndMeth=Zero  SaturateOnIntegerOverflow=on
  T-Загальний час циклу,с : Constant  Value=4.3
  V : Scope
  a : Scope
  t3 : Saturate  UpperLimit=1.15  LowerLimit=0
  Генераці1 : Subsystem  TreatAsAtomicUnit=on
  пакет2 : Subsystem
  пакет3 : Subsystem
  постійні : Subsystem
  Out1 : Outport
  Out2 : Outport  Port=2
  Out3 : Outport  Port=3
  wires:
  (t1+ t2)/1 -> t3/1
  Clock1/1 -> (t1)/1, (t1+ t2)/1, Sum1/2
  T-Загальний час циклу,с/1 -> Sum1/1
  Constant1/1 -> Генераці1/1(In1)
  Sum1/1 -> Генераці1/Trigger
  Генераці1/1(Out1) -> Switch2/2
  пакет3/1(Out1) -> Sum8/2
  пакет3/2(Out2) -> Sum9/2
  пакет2/1(Out1) -> Sum8/1
  Sum8/1 -> Switch2/3, a/1
  Switch2/1 -> Out1/1
  Sum9/1 -> Out2/1, V/1, Integrator/1
  пакет2/2(Out2) -> Sum9/1
  постійні/1(Out1) -> пакет2/3(a)
  постійні/2(Out2) -> пакет3/3(a)
  постійні/4(Out4) -> пакет3/1(ti)
  постійні/3(Out3) -> пакет2/1(ti)
  (t1)/1 -> пакет2/2(t)
  t3/1 -> пакет3/2(t)
  Integrator/1 -> Product5/2
  Product5/1 -> Scope2/1, Out3/1
  Divide/1 -> Product5/1
  Constant/1 -> Divide/1

== system model_min_mine/5 систем підйому/1/3-періодні/Пр ==
  note: (t1+t2)
  (t1) : Saturate  UpperLimit=1.15  LowerLimit=0
  Clock1 : Clock
  Constant : Constant  Value=2
  Constant1 : Constant
  Constant2 : Constant
  Constant5 : Constant
  Divide : Product  Inputs=/
  Integrator : Integrator
  Product2 : Product  SaturateOnIntegerOverflow=on  OutDataTypeStr=Inherit: Same as first input
  Product5 : Product  SaturateOnIntegerOverflow=on  OutDataTypeStr=Inherit: Same as first input
  Product6 : Product  SaturateOnIntegerOverflow=on  OutDataTypeStr=Inherit: Same as first input
  Scope2 : Scope
  Sum1 : Sum  Inputs=|+-  SaturateOnIntegerOverflow=on
  Sum2 : Sum  Inputs=|+-  SaturateOnIntegerOverflow=on
  Sum4 : Sum  Inputs=|+-  SaturateOnIntegerOverflow=on
  Sum8 : Sum  Inputs=|++  SaturateOnIntegerOverflow=on
  Sum9 : Sum  Inputs=|++  SaturateOnIntegerOverflow=on
  Switch1 : Switch  Criteria=u2 ~= 0  RndMeth=Zero  SaturateOnIntegerOverflow=on
  Switch2 : Switch  Criteria=u2 ~= 0  RndMeth=Zero  SaturateOnIntegerOverflow=on
  Switch3 : Switch  Criteria=u2 ~= 0  RndMeth=Zero  SaturateOnIntegerOverflow=on
  T-Загальний час циклу,с : Constant  Value=4.3
  V : Scope
  V1 : Scope
  ogr : Saturate  UpperLimit=100  LowerLimit=0
  t2 : DeadZone  LowerValue=0  UpperValue=3.15  SaturateOnIntegerOverflow=on
  t3 : Saturate  UpperLimit=1.15  LowerLimit=0
  Генераці : Subsystem  TreatAsAtomicUnit=on
  Генераці1 : Subsystem  TreatAsAtomicUnit=on
  Генераці2 : Subsystem  TreatAsAtomicUnit=on
  постійні : Subsystem
  Out1 : Outport
  Out2 : Outport  Port=2
  Out3 : Outport  Port=3
  wires:
  постійні/1(Out1) -> Product6/1, Switch1/3
  t2/1 -> t3/1
  t3/1 -> Product2/2
  Clock1/1 -> (t1)/1, t2/1, Sum2/1, Sum1/2
  (t1)/1 -> Product6/2, Sum4/2
  Product6/1 -> Sum9/1
  постійні/2(Out2) -> Product2/1, Switch2/1
  Product2/1 -> Sum9/2
  Sum9/1 -> ogr/1, V/1, Integrator/1
  Constant5/1 -> Генераці/1(In1)
  Sum4/1 -> Генераці/Trigger
  Генераці/1(Out1) -> Switch1/2
  Switch1/1 -> Sum8/1
  постійні/4(Out4) -> Sum4/1
  Constant1/1 -> Генераці1/1(In1)
  Sum1/1 -> Генераці1/Trigger
  Генераці1/1(Out1) -> Switch2/2
  Switch2/1 -> Sum8/2
  ogr/1 -> Out2/1
  Constant2/1 -> Генераці2/1(In1)
  Генераці2/1(Out1) -> Switch3/2
  Sum2/1 -> Генераці2/Trigger
  Sum8/1 -> Switch3/3
  Switch3/1 -> Out1/1, V1/1
  постійні/5(Out5) -> Sum1/1
  T-Загальний час циклу,с/1 -> Sum2/2
  Integrator/1 -> Product5/2
  Product5/1 -> Scope2/1, Out3/1
  Divide/1 -> Product5/1
  Constant/1 -> Divide/1

== system model_min_mine/5 систем підйому/1/4-періодна /Генераці ==
  In1 : Inport
  Trigger : TriggerPort  TriggerType=either  VariantControl=(inherit)  ShowOutputPort=on
  Out1 : Outport
  wires:
  In1/1 -> Out1/1

== system model_min_mine/5 систем підйому/1/4-періодна /Генераці1 ==
  In1 : Inport
  Trigger : TriggerPort  TriggerType=either  VariantControl=(inherit)  ShowOutputPort=on
  Out1 : Outport
  wires:
  In1/1 -> Out1/1

== system model_min_mine/5 систем підйому/1/4-періодна /Генераці2 ==
  In1 : Inport
  Trigger : TriggerPort  TriggerType=either  VariantControl=(inherit)  ShowOutputPort=on
  Out1 : Outport
  wires:
  In1/1 -> Out1/1

== system model_min_mine/5 систем підйому/1/4-періодна /Генераці3 ==
  In1 : Inport
  Trigger : TriggerPort  TriggerType=either  VariantControl=(inherit)  ShowOutputPort=on
  Out1 : Outport
  wires:
  In1/1 -> Out1/1

== system model_min_mine/5 систем підйому/1/4-періодна /постійні ==
  (t1) : Constant  Value=1.15
  (t3) : Constant  Value=2
  (t4) : Constant
  T : Constant  Value=7.15
  a1 : Constant  Value=0.5
  a3 : Constant  Value=-1
  a4 : Constant  Value=-0.95
  Out1 : Outport
  Out2 : Outport  Port=2
  Out6 : Outport  Port=3
  Out3 : Outport  Port=4
  Out4 : Outport  Port=5
  Out5 : Outport  Port=6
  Out7 : Outport  Port=7
  wires:
  a1/1 -> Out1/1
  a3/1 -> Out2/1
  (t3)/1 -> Out3/1
  (t1)/1 -> Out4/1
  (t4)/1 -> Out5/1
  a4/1 -> Out6/1
  T/1 -> Out7/1

== system model_min_mine/5 систем підйому/1/5-періодні/криво ==
  note: затримка на
      |  (t1)
  note: затримка на
      |  (t1+ t2 + t3)
  note: затримка на
      |  (t1+ t2 +t3 +t4)
  (t-2) : Saturate  UpperLimit=3.5  LowerLimit=0
  (t-4) : Saturate  UpperLimit=3.5  LowerLimit=0
  (t-5) : Saturate  LowerLimit=0
  (t1) : Saturate  LowerLimit=0
  Clock1 : Clock
      settings: Decimation=14
  Constant : Constant  Value=2
  Divide : Product  Inputs=/
  Integrator : Integrator
  Product{2..6} (5 alike) : Product  SaturateOnIntegerOverflow=on  OutDataTypeStr=Inherit: Same as first input
  Scope{1..3,5..7,9} (7 alike) : Scope
  Subsystem : Subsystem
  Subsystem1 : Subsystem
  Subsystem2 : Subsystem
  Subsystem3 : Subsystem
  Subsystem6 : Subsystem
  Sum1 : Sum  Inputs=|++++  SaturateOnIntegerOverflow=on
  Sum2 : Sum  Inputs=|++++  SaturateOnIntegerOverflow=on
  t1 : DeadZone  LowerValue=0  UpperValue=11.5  SaturateOnIntegerOverflow=on
  t2 : DeadZone  LowerValue=0  SaturateOnIntegerOverflow=on
  t5 : DeadZone  LowerValue=0  UpperValue=8  SaturateOnIntegerOverflow=on
  Допоміжний : Subsystem
  Допоміжний1 : Subsystem
  постійні : Subsystem
  Out1 : Outport
  Out2 : Outport  Port=2
  Out3 : Outport  Port=3
  wires:
  t2/1 -> (t-2)/1
  Clock1/1 -> t2/1, t5/1, t1/1, Subsystem6/2(t), Subsystem3/1(t1), Subsystem2/1(t1), (t1)/1
  постійні/5(Out5) -> Subsystem/1(t1)
  постійні/1(Out1) -> Product6/2, Subsystem/3(a1)
  (t-2)/1 -> Product4/1, Subsystem1/2(t)
  постійні/6(Out6) -> Subsystem1/1(t1)
  постійні/2(Out2) -> Product4/2, Subsystem1/3(a1)
  t5/1 -> (t-4)/1
  (t-4)/1 -> Product2/1, Допоміжний1/2(t)
  t1/1 -> (t-5)/1
  (t-5)/1 -> Product3/1
  постійні/3(Out3) -> Subsystem2/3(a1), Product2/2
  постійні/4(Out4) -> Subsystem3/3(a1), Product3/2
  Subsystem6/1(Out1) -> Out1/1, Scope1/1
  Product4/1 -> Sum1/2
  Product6/1 -> Sum1/1
  Sum1/1 -> Scope3/1, Out2/1, Integrator/1
  Subsystem/1(Out1) -> Допоміжний/1(t1), Scope5/1, Sum2/2
  (t1)/1 -> Product6/1, Subsystem/2(t), Допоміжний/2(t)
  Sum2/1 -> Subsystem6/3(a), Scope7/1
  постійні/9(Out9) -> Subsystem6/1(Сума t)
  Product2/1 -> Sum1/3, Scope6/1
  Product3/1 -> Sum1/4
  Subsystem3/1(Out1) -> Scope9/1, Sum2/4
  Subsystem1/1(Out1) -> Допоміжний/3(a1)
  Допоміжний/1(Out1) -> Sum2/1
  постійні/10(Out10) -> Subsystem2/2(t)
  Subsystem2/1(Out1) -> Допоміжний1/3(a1)
  Допоміжний1/1(Out1) -> Sum2/3
  постійні/7(Out7) -> Допоміжний1/1(t1)
  постійні/8(Out8) -> Subsystem3/2(t)
  Integrator/1 -> Product5/2
  Product5/1 -> Scope2/1, Out3/1
  Divide/1 -> Product5/1
  Constant/1 -> Divide/1

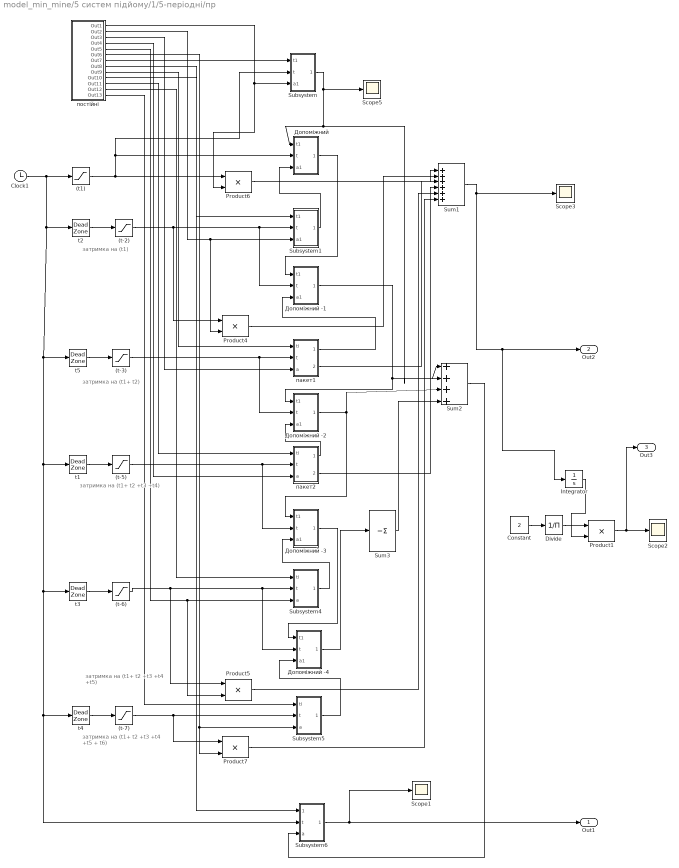
== system model_min_mine/5 систем підйому/1/5-періодні/пр ==
  note: затримка на
      |  (t1)
  note: затримка на
      |  (t1+ t2)
  note: затримка на
      |  (t1+ t2 +t3 +t4)
  note: затримка на
      |  (t1+ t2 +t3 +t4 +t5)
  note: затримка на
      |  (t1+ t2 +t3 +t4 +t5 + t6)
  (t-2) : Saturate  UpperLimit=3.5  LowerLimit=0
  (t-3) : Saturate  LowerLimit=0
  (t-5) : Saturate  LowerLimit=0
  (t-6) : Saturate  UpperLimit=3.5  LowerLimit=0
  (t-7) : Saturate  LowerLimit=0
  (t1) : Saturate  LowerLimit=0
  Clock1 : Clock
      settings: Decimation=14
  Constant : Constant  Value=2
  Divide : Product  Inputs=/
  Integrator : Integrator
  Product{1,4..7} (5 alike) : Product  SaturateOnIntegerOverflow=on  OutDataTypeStr=Inherit: Same as first input
  Scope{1..3,5} (4 alike) : Scope
  Subsystem : Subsystem
  Subsystem1 : Subsystem
  Subsystem4 : Subsystem
  Subsystem5 : Subsystem
  Subsystem6 : Subsystem
  Sum1 : Sum  Inputs=|++++++  SaturateOnIntegerOverflow=on
  Sum2 : Sum  Inputs=|++++  SaturateOnIntegerOverflow=on
  Sum3 : Sum  Inputs=-  SaturateOnIntegerOverflow=on
  t1 : DeadZone  LowerValue=0  UpperValue=7.5  SaturateOnIntegerOverflow=on
  t2 : DeadZone  LowerValue=0  SaturateOnIntegerOverflow=on
  t3 : DeadZone  LowerValue=0  UpperValue=8  SaturateOnIntegerOverflow=on
  t4 : DeadZone  LowerValue=0  UpperValue=11.5  SaturateOnIntegerOverflow=on
  t5 : DeadZone  LowerValue=0  UpperValue=4  SaturateOnIntegerOverflow=on
  Допоміжний : Subsystem
  Допоміжний -1 : Subsystem
  Допоміжний -2 : Subsystem
  Допоміжний -3 : Subsystem
  Допоміжний -4 : Subsystem
  пакет1 : Subsystem
  пакет2 : Subsystem
  постійні : Subsystem
  Out1 : Outport
  Out2 : Outport  Port=2
  Out3 : Outport  Port=3
  wires:
  t2/1 -> (t-2)/1
  Clock1/1 -> t2/1, t5/1, t1/1, t3/1, Subsystem6/2(t), t4/1, (t1)/1
  постійні/7(Out7) -> Subsystem/1(t1)
  постійні/1(Out1) -> Product6/2, Subsystem/3(a1)
  (t-2)/1 -> Product4/1, Subsystem1/2(t), Допоміжний -1/2(t)
  постійні/8(Out8) -> Subsystem1/1(t1)
  постійні/2(Out2) -> Product4/2, Subsystem1/3(a1)
  t5/1 -> (t-3)/1
  (t-3)/1 -> пакет1/2(t), Допоміжний -2/2(t)
  t1/1 -> (t-5)/1
  (t-5)/1 -> пакет2/2(t), Допоміжний -3/2(t)
  постійні/9(Out9) -> пакет1/1(ti)
  постійні/11(Out11) -> пакет2/1(ti)
  постійні/3(Out3) -> пакет1/3(a)
  постійні/4(Out4) -> пакет2/3(a)
  t3/1 -> (t-6)/1
  (t-6)/1 -> Product5/1, Subsystem4/2(t), Допоміжний -4/2(t)
  постійні/12(Out12) -> Subsystem4/1(ti)
  постійні/5(Out5) -> Subsystem4/3(a), Product5/2
  t4/1 -> (t-7)/1
  (t-7)/1 -> Subsystem5/2(t), Product7/1
  постійні/13(Out13) -> Subsystem5/1(ti)
  постійні/6(Out6) -> Product7/2, Subsystem5/3(a)
  постійні/10(Out10) -> Subsystem6/1(Сума t)
  Subsystem6/1(Out1) -> Out1/1, Scope1/1
  Product4/1 -> Sum1/2
  Product6/1 -> Sum1/1
  пакет1/2(Out2) -> Sum1/3
  пакет2/2(Out2) -> Sum1/4
  Product5/1 -> Sum1/5
  Product7/1 -> Sum1/6
  Sum1/1 -> Scope3/1, Out2/1, Integrator/1
  Subsystem/1(Out1) -> Допоміжний/1(t1), Sum2/2, Scope5/1
  (t1)/1 -> Product6/1, Subsystem/2(t), Допоміжний/2(t)
  Subsystem1/1(Out1) -> Допоміжний/3(a1)
  Допоміжний/1(Out1) -> Допоміжний -1/1(t1)
  пакет1/1(Out1) -> Допоміжний -1/3(a1)
  Допоміжний -1/1(Out1) -> Допоміжний -2/1(t1), Sum2/1
  пакет2/1(Out1) -> Допоміжний -2/3(a1)
  Допоміжний -2/1(Out1) -> Допоміжний -3/1(t1), Sum2/3
  Subsystem4/1(Out1) -> Допоміжний -3/3(a1)
  Допоміжний -3/1(Out1) -> Допоміжний -4/1(t1)
  Subsystem5/1(Out1) -> Допоміжний -4/3(a1)
  Sum2/1 -> Subsystem6/3(a)
  Допоміжний -4/1(Out1) -> Sum3/1
  Sum3/1 -> Sum2/4
  Integrator/1 -> Product1/2
  Product1/1 -> Scope2/1, Out3/1
  Divide/1 -> Product1/1
  Constant/1 -> Divide/1

== system model_min_mine/5 систем підйому/1/6-періодні/6-ти періодна криволінійна ==
  note: затримка на
      |  (t1)
  note: затримка на
      |  (t1+ t2 + t3)
  note: затримка на
      |  (t1+ t2 +t3 +t4 +t4/)
  (t-2) : Saturate  UpperLimit=3.5  LowerLimit=0
  (t-4) : Saturate  UpperLimit=3.5  LowerLimit=0
  (t-5) : Saturate  LowerLimit=0
  (t1) : Saturate  LowerLimit=0
  Clock1 : Clock
      settings: Decimation=14
  Constant : Constant  Value=2
  Divide : Product  Inputs=/
  Integrator : Integrator
  Product3 : Product  SaturateOnIntegerOverflow=on  OutDataTypeStr=Inherit: Same as first input
  Product5 : Product  SaturateOnIntegerOverflow=on  OutDataTypeStr=Inherit: Same as first input
  Product6 : Product  SaturateOnIntegerOverflow=on  OutDataTypeStr=Inherit: Same as first input
  Scope{1..3,5,7,9} (6 alike) : Scope
  Scope6 : Scope  NumInputPorts=3
  Subsystem : Subsystem
  Subsystem3 : Subsystem
  Subsystem6 : Subsystem
  Sum1 : Sum  Inputs=|++++  SaturateOnIntegerOverflow=on
  Sum2 : Sum  Inputs=|++++  SaturateOnIntegerOverflow=on
  t1 : DeadZone  LowerValue=0  UpperValue=12  SaturateOnIntegerOverflow=on
  t2 : DeadZone  LowerValue=0  SaturateOnIntegerOverflow=on
  t5 : DeadZone  LowerValue=0  UpperValue=8  SaturateOnIntegerOverflow=on
  Допоміжний : Subsystem
  Допоміжний1 : Subsystem
  пакет1 : Subsystem
  пакет2 : Subsystem
  постійні : Subsystem
  Out1 : Outport
  Out2 : Outport  Port=2
  Out3 : Outport  Port=3
  wires:
  t2/1 -> (t-2)/1
  Clock1/1 -> (t1)/1, t2/1, t5/1, t1/1, Subsystem6/2(t), Subsystem3/1(t1)
  постійні/5(Out5) -> Subsystem/1(t1)
  постійні/1(Out1) -> Product6/2, Subsystem/3(a1)
  (t-2)/1 -> пакет1/2(t)
  постійні/6(Out6) -> пакет1/1(ti)
  постійні/2(Out2) -> пакет1/3(a)
  t5/1 -> (t-4)/1
  (t-4)/1 -> Допоміжний1/2(t), пакет2/2(t)
  t1/1 -> (t-5)/1
  (t-5)/1 -> Product3/1
  постійні/3(Out3) -> пакет2/3(a)
  постійні/4(Out4) -> Subsystem3/3(a1), Product3/2
  Subsystem6/1(Out1) -> Out1/1, Scope1/1
  Product6/1 -> Sum1/1
  Sum1/1 -> Scope3/1, Out2/1, Scope6/2, Integrator/1
  Subsystem/1(Out1) -> Допоміжний/1(t1), Scope5/1, Sum2/2
  (t1)/1 -> Product6/1, Subsystem/2(t), Допоміжний/2(t)
  Sum2/1 -> Subsystem6/3(a), Scope7/1
  постійні/9(Out9) -> Subsystem6/1(Сума t)
  Product3/1 -> Sum1/4
  Subsystem3/1(Out1) -> Scope9/1, Sum2/4, Scope6/3
  пакет1/1(Out1) -> Допоміжний/3(a1)
  Допоміжний/1(Out1) -> Sum2/1
  пакет2/1(Out1) -> Допоміжний1/3(a1)
  Допоміжний1/1(Out1) -> Sum2/3, Scope6/1
  постійні/7(Out7) -> Допоміжний1/1(t1), пакет2/1(ti)
  постійні/8(Out8) -> Subsystem3/2(t)
  пакет1/2(Out2) -> Sum1/2
  пакет2/2(Out2) -> Sum1/3
  Integrator/1 -> Product5/2
  Product5/1 -> Scope2/1, Out3/1
  Divide/1 -> Product5/1
  Constant/1 -> Divide/1

== system model_min_mine/5 систем підйому/1/6-періодні/6-ти періодна пр ==
  note: затримка на
      |  (t1)
  note: затримка на
      |  (t1+ t2 + t3)
  note: затримка на
      |  (t1+ t2 +t3 +t4 +t4/)
  (t-2) : Saturate  UpperLimit=3.5  LowerLimit=0
  (t-4) : Saturate  UpperLimit=3.5  LowerLimit=0
  (t-5) : Saturate  LowerLimit=0
  (t1) : Saturate  LowerLimit=0
  Clock1 : Clock
      settings: Decimation=14
  Constant : Constant  Value=2
  Divide : Product  Inputs=/
  Integrator : Integrator
  Product{2..6} (5 alike) : Product  SaturateOnIntegerOverflow=on  OutDataTypeStr=Inherit: Same as first input
  Scope{1..3,5,7,9} (6 alike) : Scope
  Scope6 : Scope  NumInputPorts=3
  Subsystem : Subsystem
  Subsystem1 : Subsystem
  Subsystem2 : Subsystem
  Subsystem3 : Subsystem
  Subsystem6 : Subsystem
  Sum1 : Sum  Inputs=|++++  SaturateOnIntegerOverflow=on
  Sum2 : Sum  Inputs=|++++  SaturateOnIntegerOverflow=on
  t1 : DeadZone  LowerValue=0  UpperValue=12  SaturateOnIntegerOverflow=on
  t2 : DeadZone  LowerValue=0  SaturateOnIntegerOverflow=on
  t5 : DeadZone  LowerValue=0  UpperValue=8  SaturateOnIntegerOverflow=on
  Допоміжний : Subsystem
  Допоміжний1 : Subsystem
  постійні : Subsystem
  Out1 : Outport
  Out2 : Outport  Port=2
  Out3 : Outport  Port=3
  wires:
  t2/1 -> (t-2)/1
  Clock1/1 -> t2/1, t5/1, t1/1, Subsystem6/2(t), Subsystem3/1(t1), Subsystem2/1(t1), (t1)/1
  постійні/5(Out5) -> Subsystem/1(t1)
  постійні/1(Out1) -> Product6/2, Subsystem/3(a1)
  (t-2)/1 -> Product4/1, Subsystem1/2(t)
  постійні/6(Out6) -> Subsystem1/1(t1)
  постійні/2(Out2) -> Product4/2, Subsystem1/3(a1)
  t5/1 -> (t-4)/1
  (t-4)/1 -> Product2/1, Допоміжний1/2(t)
  t1/1 -> (t-5)/1
  (t-5)/1 -> Product3/1
  постійні/3(Out3) -> Subsystem2/3(a1), Product2/2
  постійні/4(Out4) -> Subsystem3/3(a1), Product3/2
  Subsystem6/1(Out1) -> Out1/1, Scope1/1
  Product4/1 -> Sum1/2
  Product6/1 -> Sum1/1
  Sum1/1 -> Scope3/1, Out2/1, Scope6/2, Integrator/1
  Subsystem/1(Out1) -> Допоміжний/1(t1), Scope5/1, Sum2/2
  (t1)/1 -> Product6/1, Subsystem/2(t), Допоміжний/2(t)
  Sum2/1 -> Subsystem6/3(a), Scope7/1
  постійні/9(Out9) -> Subsystem6/1(Сума t)
  Product2/1 -> Sum1/3
  Product3/1 -> Sum1/4
  Subsystem3/1(Out1) -> Scope9/1, Sum2/4, Scope6/3
  Subsystem1/1(Out1) -> Допоміжний/3(a1)
  Допоміжний/1(Out1) -> Sum2/1
  постійні/10(Out10) -> Subsystem2/2(t)
  Subsystem2/1(Out1) -> Допоміжний1/3(a1)
  Допоміжний1/1(Out1) -> Sum2/3, Scope6/1
  постійні/7(Out7) -> Допоміжний1/1(t1)
  постійні/8(Out8) -> Subsystem3/2(t)
  Integrator/1 -> Product5/2
  Product5/1 -> Scope2/1, Out3/1
  Divide/1 -> Product5/1
  Constant/1 -> Divide/1
